simulink model "TGASMODEL"  (R2021b)
settings: Solver=VariableStepAuto  StartTime=0.0  StopTime=simstoptime  RelTol=1e-3
values from neighbouring files (symbols this model uses):
  initial_lane = 0    [setupscript.m]
  Ts = 0.1    [setupscript.m]
  v_set = 33    [setupscript.m]
  VB = 30.5556    [setupscript.m]
  velocity_left_lane_max = 35    [setupscript.m]
  velocity_right_lane_max = 35    [setupscript.m]
undefined symbols (not defined in the file or in its folder): driving
libraries: drivingscenarioandsensors x3, autolibshared x1
settings Model: Creator=Milin  LastModifiedBy=Milin.Patel
settings SolverCC: AlgebraicLoopSolver=TrustRegion
settings DebuggingCC: ParameterPrecisionLossMsg=none  SFMachineParentedDataDiag=warning

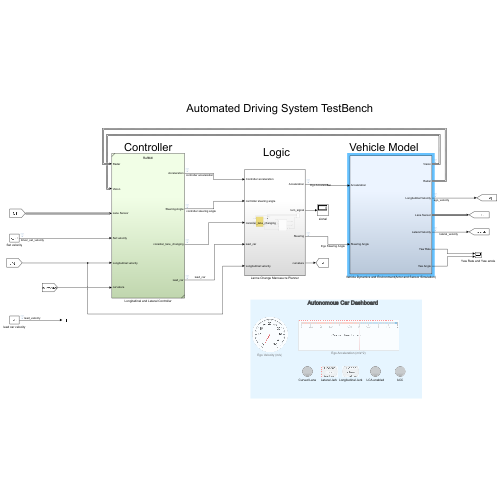
[thumbnail: Simulink's stored preview of the top-level diagram]
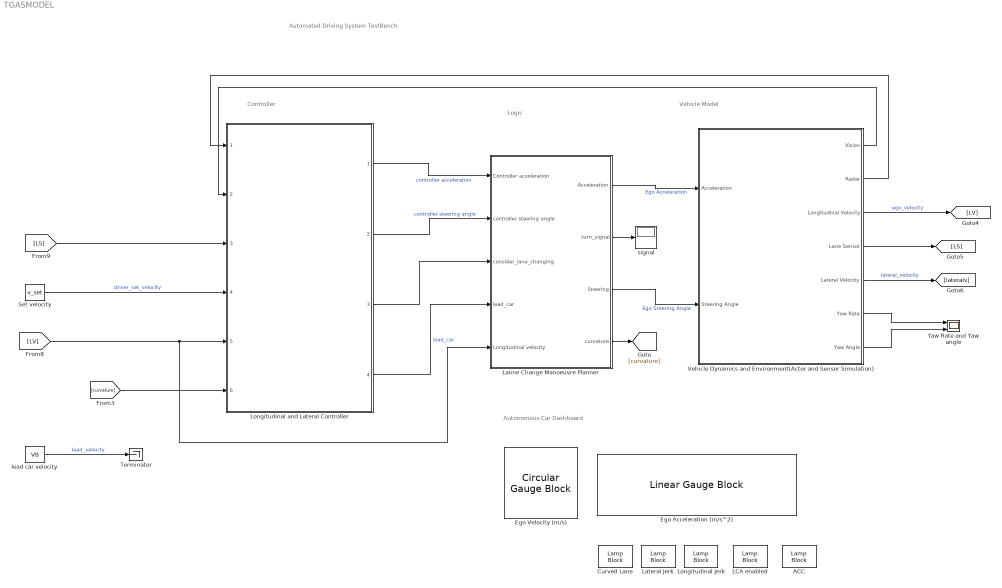
== system TGASMODEL ==
  note: Autonomous Car Dashboard
  note: Automated Driving System TestBench
  note: Controller
  note: Vehicle Model
  note: Logic
  ACC : LampBlock  LabelPosition=Hide
  Curved Lane : LampBlock  LabelPosition=Hide
  Ego Acceleration (m/s^2) : LinearGaugeBlock  LabelPosition=Hide  ScaleMin=-3  ScaleMax=2
  Ego Velocity (m/s) : CircularGaugeBlock  LabelPosition=Hide  ScaleMax=50  TickInterval=5
  LCA enabled : LampBlock  LabelPosition=Hide
  Lanne Change Manoeuvre Planner : Subsystem
  Lateral Jerk : LampBlock  LabelPosition=Hide
  Longitudinal Jerk : LampBlock  LabelPosition=Hide
  Longitudinal and Lateral Controller : Subsystem  ReferencedSubsystem=RefMdl
  Set velocity : Constant  Value=v_set  SampleTime=Ts
  Terminator : Terminator
  Vehicle Dynamics and Environment(Actor and Sensor Simulation) : Subsystem
  Yaw Rate and Yaw angle : Scope  NumInputPorts=2
  lead car velocity : Constant  Value=VB  SampleTime=Ts
  signal : Display
  wires:
  Vehicle Dynamics and Environment(Actor and Sensor Simulation)/3(Longitudinal Velocity) -> [LV]  "ego_velocity"
  Vehicle Dynamics and Environment(Actor and Sensor Simulation)/7(Yaw Angle) -> Yaw Rate and Yaw angle/2
  Vehicle Dynamics and Environment(Actor and Sensor Simulation)/4(Lane Sensor) -> [LS]
  Longitudinal and Lateral Controller/2 -> Lanne Change Manoeuvre Planner/2(controller steering angle)  "controller steering angle"
  Lanne Change Manoeuvre Planner/1(Acceleration) -> Vehicle Dynamics and Environment(Actor and Sensor Simulation)/1(Acceleration)  "Ego Acceleration"
  Vehicle Dynamics and Environment(Actor and Sensor Simulation)/6(Yaw Rate) -> Yaw Rate and Yaw angle/1
  Lanne Change Manoeuvre Planner/2(turn_signal) -> signal/1
  Vehicle Dynamics and Environment(Actor and Sensor Simulation)/1(Vision) -> Longitudinal and Lateral Controller/2
  Vehicle Dynamics and Environment(Actor and Sensor Simulation)/2(Radar) -> Longitudinal and Lateral Controller/1
  [LS] -> Longitudinal and Lateral Controller/3
  Longitudinal and Lateral Controller/3 -> Lanne Change Manoeuvre Planner/3(consider_lane_changing)
  Lanne Change Manoeuvre Planner/4(curvature) -> [curvature]
  Lanne Change Manoeuvre Planner/3(Steering) -> Vehicle Dynamics and Environment(Actor and Sensor Simulation)/2(Steering Angle)  "Ego Steering Angle"
  [curvature] -> Longitudinal and Lateral Controller/6
  Set velocity/1 -> Longitudinal and Lateral Controller/4  "driver_set_velocity"
  Longitudinal and Lateral Controller/1 -> Lanne Change Manoeuvre Planner/1(Controller acceleration)  "controller acceleration"
  Vehicle Dynamics and Environment(Actor and Sensor Simulation)/5(Lateral Velocity) -> [lateralv]  "lateral_velocity"
  [LV] -> Lanne Change Manoeuvre Planner/5(Longitudinal velocity), Longitudinal and Lateral Controller/5
  lead car velocity/1 -> Terminator/1  "lead_velocity"
  Longitudinal and Lateral Controller/4 -> Lanne Change Manoeuvre Planner/4(lead_car)  "lead_car"

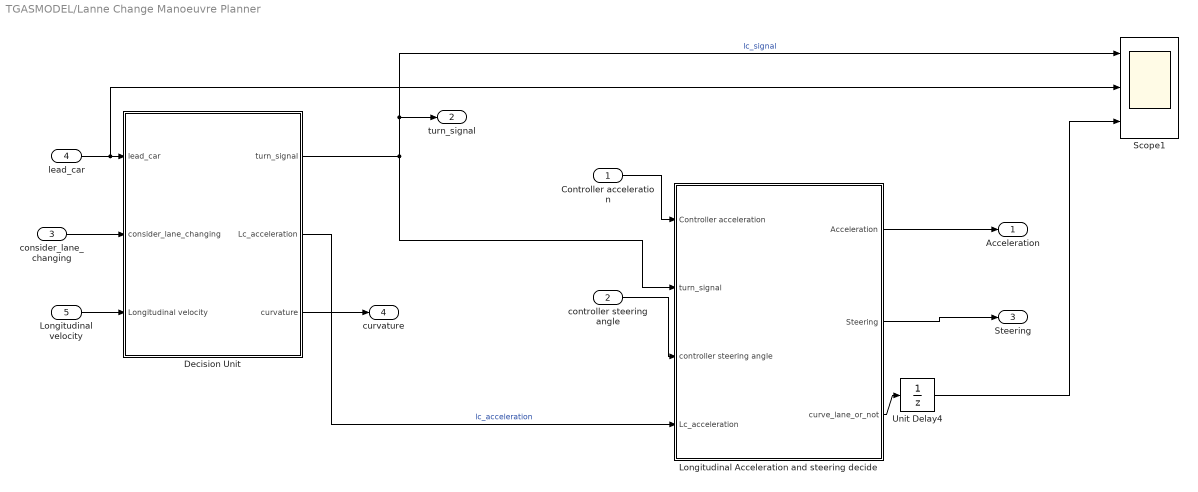
== system TGASMODEL/Lanne Change Manoeuvre Planner ==
  Controller acceleration : Inport
  controller steering angle : Inport  Port=2
  consider_lane_changing : Inport  Port=3
  lead_car : Inport  Port=4
  Longitudinal velocity : Inport  Port=5
  Decision Unit : Subsystem
  Longitudinal Acceleration and steering decide : Subsystem
  Scope1 : Scope  NumInputPorts=3
  Unit Delay4 : UnitDelay  SampleTime=-1  HasFrameUpgradeWarning=on
  Acceleration : Outport
  turn_signal : Outport  Port=2
  Steering : Outport  Port=3
  curvature : Outport  Port=4
  wires:
  consider_lane_changing/1 -> Decision Unit/2(consider_lane_changing)
  controller steering angle/1 -> Longitudinal Acceleration and steering decide/3(controller steering angle)
  Controller acceleration/1 -> Longitudinal Acceleration and steering decide/1(Controller acceleration)
  Longitudinal velocity/1 -> Decision Unit/3(Longitudinal velocity)
  lead_car/1 -> Scope1/2, Decision Unit/1(lead_car)
  Decision Unit/1(turn_signal) -> Scope1/1, turn_signal/1, Longitudinal Acceleration and steering decide/2(turn_signal)  "lc_signal"
  Decision Unit/3(curvature) -> curvature/1
  Decision Unit/2(Lc_acceleration) -> Longitudinal Acceleration and steering decide/4(Lc_acceleration)  "lc_acceleration"
  Longitudinal Acceleration and steering decide/1(Acceleration) -> Acceleration/1
  Longitudinal Acceleration and steering decide/2(Steering) -> Steering/1
  Unit Delay4/1 -> Scope1/3
  Longitudinal Acceleration and steering decide/3(curve_lane_or_not) -> Unit Delay4/1

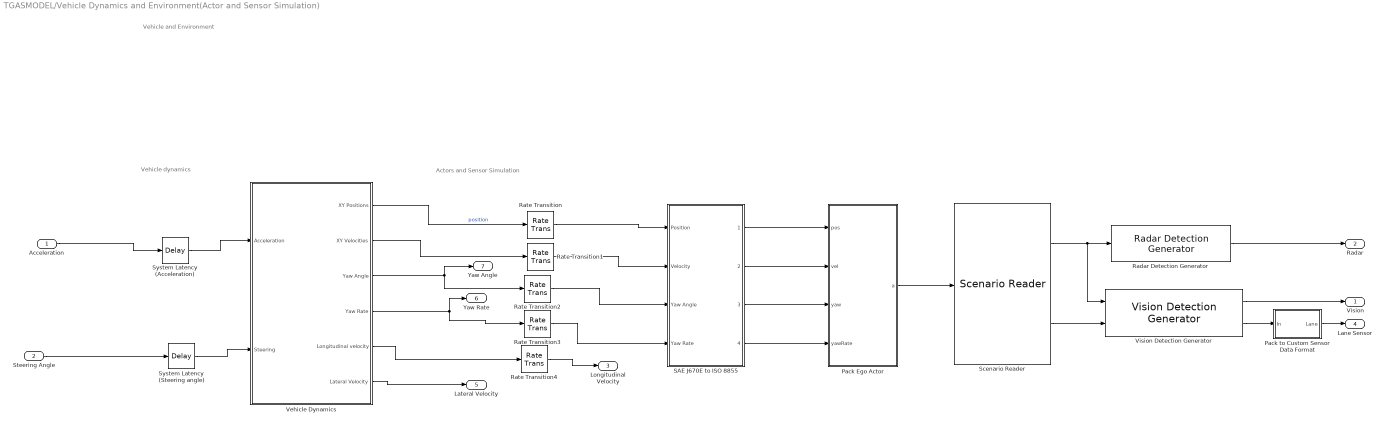
== system TGASMODEL/Vehicle Dynamics and Environment(Actor and Sensor Simulation) ==
  note: Vehicle dynamics
  note: Actors and Sensor Simulation
  note: Vehicle and Environment
  Acceleration : Inport  Unit=m/s^2
  Steering Angle : Inport  Port=2  Unit=rad
  Pack Ego Actor : MATLAB Function  TreatAsAtomicUnit=on
  Pack to Custom Sensor Data Format : Subsystem
  Radar Detection Generator : drivingscenarioandsensors/Radar Detection Generator  SensorIndex=2  UpdateInterval=0.1  SensorLocation=[ 3.7, 0 ]  Height=0.2  Yaw=0  Pitch=0  Roll=0  BusNameSource=Property  BusName=BusRadar  MaxNumDetectionsSource=Property  MaxNumDetections=50  DetectionCoordinates=Ego Cartesian  SimulateUsing=Interpreted execution  AzimuthResolution=4  ElevationResolution=10  RangeResolution=2.5  RangeRateResolution=0.5  AzimuthBiasFraction=0.1  ElevationBiasFraction=0.1  RangeBiasFraction=0.05  RangeRateBiasFraction=0.05  FieldOfView=[ 20, 5 ]  MaxRange=174  RangeRateLimits=[ -100, 100 ]  DetectionProbability=0.9  FalseAlarmRate=1e-6  ReferenceRange=100  ReferenceRCS=0  HasElevation=off  HasRangeRate=on  HasNoise=on  HasFalseAlarms=on  HasOcclusion=on  InitialSeedSource=Repeatable  InitialSeed=0  UsedSeed=driving.internal.SimulinkUtilities.seedManager(gcb)  ActorProfilesSource=MATLAB expression  ActorProfilesParameters=driving.internal.ActorProfilesRadarParameters  ActorProfilesExpression=actor_Profiles
      settings: SourceProductBaseCode=DR
  Rate Transition{,1..4} (5 alike) : RateTransition  OutPortSampleTime=Ts
  SAE J670E to ISO 8855 : Subsystem
  Scenario Reader : drivingscenarioandsensors/Scenario Reader  ScenarioSource=From file  ScenarioFileName=D:\Simulations\Thesis submission digital files\Thesis submission digital files\TGAS Model Testbench\customlc.mat  ScenarioVariableName=scenario  OutputCoordinateSystem=Vehicle coordinates  EgoVehicleSource=Input port  EgoVehicleActorID=1  OrientVehiclesOnRoad=off  OutputEgoVehiclePose=off  OutputEgoVehicleState=off  SampleTime=0.1  LaneBoundaryOutput=Ego vehicle lane boundaries  LaneBoundaryDistance=0:0.5:60  LaneBoundaryLocation=Inner edge of lane markings  BusNameSource=Auto  BusName=BusActors1  BusNumActorsSource=Scenario  BusNumActors=100  BusName2Source=Auto  BusName2=BusLaneBoundaries  BusNumLaneBoundariesSource=Scenario  BusNumLaneBoundaries=10  BusName3Source=Auto  BusName3=BusEgoActor  BusName4Source=Auto  BusName4=BusEgoState  ShowCoordinateLabels=on  SimulateUsing=Interpreted execution
  System Latency (Acceleration) : TransportDelay  DelayTime=Ts  BufferSize=2048
  System Latency (Steering angle) : TransportDelay  DelayTime=Ts  BufferSize=2048
  Vehicle Dynamics : Subsystem  VariantControl=Variant2
  Vision Detection Generator : drivingscenarioandsensors/Vision Detection Generator  SensorIndex=1  DetectorOutput=Lanes and objects  UpdateInterval=0.1  LaneUpdateInterval=0.1  SensorLocation=[ 1.9, 0 ]  Height=1.1  Yaw=0  Pitch=1  Roll=0  BusNameSource=Property  BusName=BusVision  BusName2Source=Property  BusName2=BusLanes  MaxNumDetectionsSource=Property  MaxNumDetections=20  MaxNumLanesSource=Property  MaxNumLanes=2  DetectionCoordinates=Ego Cartesian  SimulateUsing=Interpreted execution  MaxRange=150  BoundingBoxAccuracy=5  ProcessNoiseIntensity=5  MaxSpeed=50  MaxAllowedOcclusion=0.5  MinObjectImageSize=[ 10, 10 ]  DetectionProbability=0.9  FalsePositivesPerImage=0.1  MinLaneImageSize=[ 20, 3 ]  LaneBoundaryAccuracy=3  HasNoise=on  InitialSeedSource=Repeatable  InitialSeed=0  UsedSeed=driving.internal.SimulinkUtilities.seedManager(gcb)  ActorProfilesSource=MATLAB expression  ActorProfilesParameters=driving.internal.ActorProfilesParameters  ActorProfilesExpression=actor_Profiles  Intrinsics=driving.internal.cameraIntrinsics('FocalLength',[ 800,800 ])
  Vision : Outport  VectorParamsAs1DForOutWhenUnconnected=off
  Radar : Outport  Port=2  VectorParamsAs1DForOutWhenUnconnected=off
  Longitudinal Velocity : Outport  Port=3  VectorParamsAs1DForOutWhenUnconnected=off
  Lane Sensor : Outport  Port=4  VectorParamsAs1DForOutWhenUnconnected=off
  Lateral Velocity : Outport  Port=5  VectorParamsAs1DForOutWhenUnconnected=off
  Yaw Rate : Outport  Port=6
  Yaw Angle : Outport  Port=7
  wires:
  Scenario Reader/1 -> Vision Detection Generator/1, Radar Detection Generator/1
  Vehicle Dynamics/2(XY Velocities) -> Rate Transition1/1
  Vehicle Dynamics/1(XY Positions) -> Rate Transition/1  "position"
  Scenario Reader/2 -> Vision Detection Generator/2
  Vision Detection Generator/1 -> Vision/1
  Radar Detection Generator/1 -> Radar/1
  Pack Ego Actor/1(a) -> Scenario Reader/1
  Acceleration/1 -> System Latency (Acceleration)/1
  Steering Angle/1 -> System Latency (Steering angle)/1
  System Latency (Acceleration)/1 -> Vehicle Dynamics/1(Acceleration)
  System Latency (Steering angle)/1 -> Vehicle Dynamics/2(Steering)
  SAE J670E to ISO 8855/1(1) -> Pack Ego Actor/1(pos)
  SAE J670E to ISO 8855/2(2) -> Pack Ego Actor/2(vel)
  SAE J670E to ISO 8855/3(3) -> Pack Ego Actor/3(yaw)
  SAE J670E to ISO 8855/4(4) -> Pack Ego Actor/4(yawRate)
  Rate Transition3/1 -> SAE J670E to ISO 8855/4(Yaw Rate)
  Rate Transition2/1 -> SAE J670E to ISO 8855/3(Yaw Angle)
  Rate Transition1/1 -> SAE J670E to ISO 8855/2(Velocity)
  Rate Transition/1 -> SAE J670E to ISO 8855/1(Position)
  Vehicle Dynamics/6(Lateral Velocity) -> Lateral Velocity/1
  Vehicle Dynamics/3(Yaw Angle) -> Yaw Angle/1, Rate Transition2/1
  Vehicle Dynamics/4(Yaw Rate) -> Yaw Rate/1, Rate Transition3/1
  Vehicle Dynamics/5(Longitudinal velocity) -> Rate Transition4/1
  Rate Transition4/1 -> Longitudinal Velocity/1
  Vision Detection Generator/2 -> Pack to Custom Sensor Data Format/1(In)
  Pack to Custom Sensor Data Format/1("Lane ") -> Lane Sensor/1

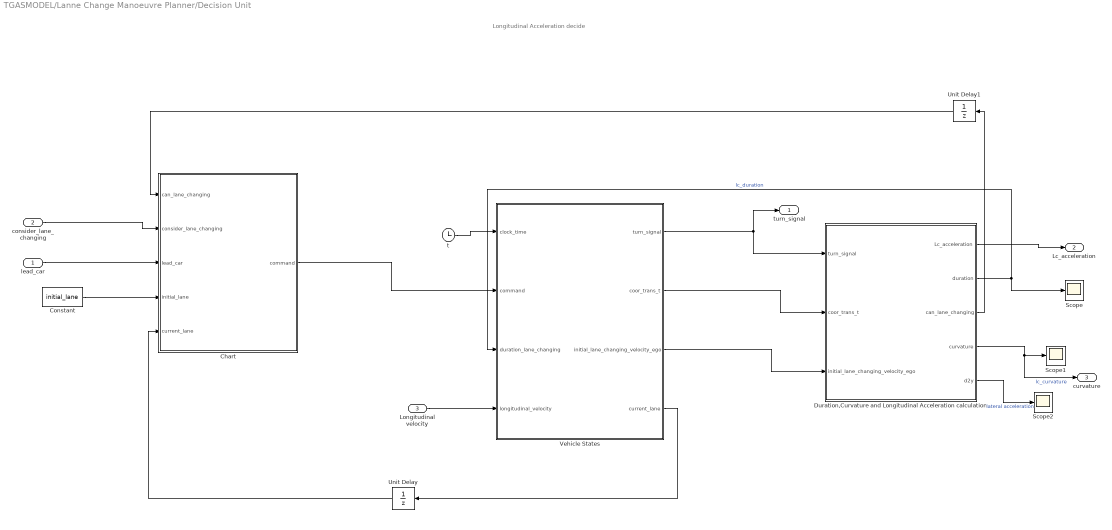
== system TGASMODEL/Lanne Change Manoeuvre Planner/Decision Unit ==
  note: Longitudinal Acceleration decide
  lead_car : Inport
  consider_lane_changing : Inport  Port=2
  Longitudinal velocity : Inport  Port=3
  Chart : Stateflow chart  TreatAsAtomicUnit=on
  Constant : Constant  Value=initial_lane
  Duration,Curvature and Longitudinal Acceleration calculation : Subsystem
  Scope : Scope
  Scope1 : Scope
  Scope2 : Scope
  Unit Delay : UnitDelay  SampleTime=-1  HasFrameUpgradeWarning=on
  Unit Delay1 : UnitDelay  SampleTime=-1  HasFrameUpgradeWarning=on
  Vehicle States : Stateflow chart  TreatAsAtomicUnit=on
      settings: PortSchema="{\"entries\":[{\"content\":{\"sides\":[{\"content\":{\"connectorIds\":[\"In2\",\"In1\",\"In3\",\"In4\"]},\"type\":\"ConnectorPlacement.EquallySpacedRectSide\",\"uuid\":\"633906ca-579d-4042-9cc9-7aca433b340e\"},{\"content\":{\"connectorIds\":[\"Out1\",\"Out2\",\"Out3\",\"Out4\"],\"side\":\"RIGHT\"},\"type\":\"ConnectorPlacement.EquallySpacedRectSide\",\"uuid\":\"b2f4b13f-832c-4f85-a2c3-5544fdd2b38b\"},{\"content\":{\"connectorIds\":[],\"side\":\"TOP\"},\"type\":\"ConnectorPlacement.EquallySpacedRectSide\",\"uuid\":\"a13a6fde-8974-48e1-9856-53eff330f07d\"}]},\"type\":\"ConnectorPlacement.EquallySpacedConnector\",\"uuid\":\"3aa8cc94-316d-4e92-871e-4708a17b4e4c\"}],\"packageUris\":[\"http://schema.mathworks.com/mf0/Connector/R2020b\"],\"version\":\"1.0\"}"
  t : Clock
  turn_signal : Outport
  Lc_acceleration : Outport  Port=2
  curvature : Outport  Port=3
  wires:
  Vehicle States/1(turn_signal) -> Duration,Curvature and Longitudinal Acceleration calculation/1(turn_signal), turn_signal/1
  t/1 -> Vehicle States/2(clock_time)
  Vehicle States/3(initial_lane_changing_velocity_ego) -> Duration,Curvature and Longitudinal Acceleration calculation/3(initial_lane_changing_velocity_ego)
  Duration,Curvature and Longitudinal Acceleration calculation/1(Lc_acceleration) -> Lc_acceleration/1
  Duration,Curvature and Longitudinal Acceleration calculation/2(duration) -> Scope/1, Vehicle States/3(duration_lane_changing)  "lc_duration"
  Duration,Curvature and Longitudinal Acceleration calculation/4(curvature) -> curvature/1, Scope1/1  "lc_curvature"
  Longitudinal velocity/1 -> Vehicle States/4(longitudinal_velocity)
  Vehicle States/2(coor_trans_t) -> Duration,Curvature and Longitudinal Acceleration calculation/2(coor_trans_t)
  lead_car/1 -> Chart/3(lead_car)
  consider_lane_changing/1 -> Chart/2(consider_lane_changing)
  Constant/1 -> Chart/4(initial_lane)
  Chart/1(command) -> Vehicle States/1(command)
  Vehicle States/4(current_lane) -> Unit Delay/1
  Unit Delay/1 -> Chart/5(current_lane)
  Duration,Curvature and Longitudinal Acceleration calculation/3(can_lane_changing) -> Unit Delay1/1
  Unit Delay1/1 -> Chart/1(can_lane_changing)
  Duration,Curvature and Longitudinal Acceleration calculation/5(d2y) -> Scope2/1  "lateral acceleration"

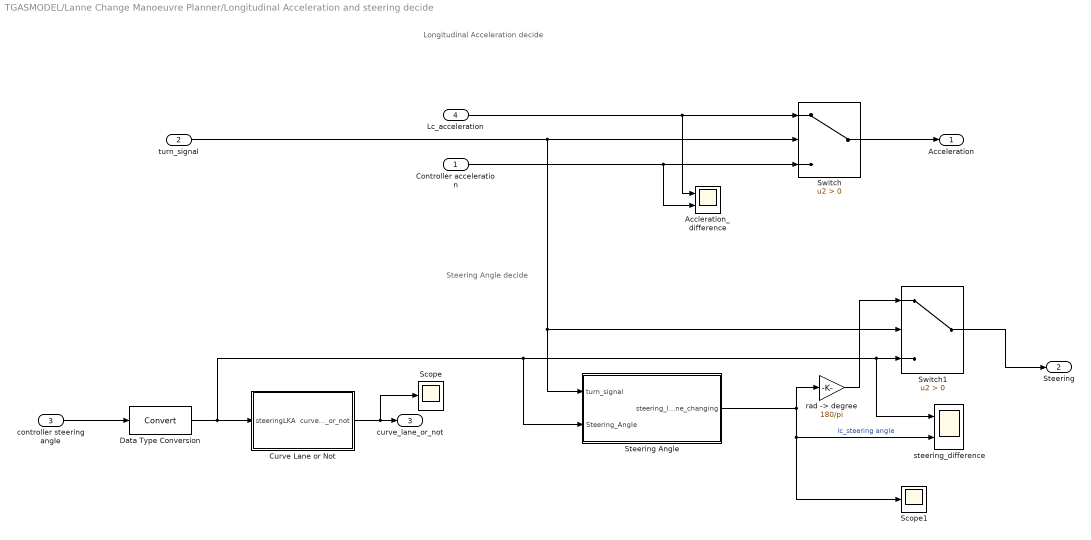
== system TGASMODEL/Lanne Change Manoeuvre Planner/Longitudinal Acceleration and steering decide ==
  note: Steering Angle decide
  note: Longitudinal Acceleration decide
  Controller acceleration : Inport
  turn_signal : Inport  Port=2
  controller steering angle : Inport  Port=3
  Lc_acceleration : Inport  Port=4
  Accleration_difference : Scope  NumInputPorts=2
  Curve Lane or Not : MATLAB Function  TreatAsAtomicUnit=on
  Data Type Conversion : DataTypeConversion
  Scope : Scope
  Scope1 : Scope
  "Steering Angle " : MATLAB Function  TreatAsAtomicUnit=on
  Switch : Switch  Criteria=u2 > Threshold
  Switch1 : Switch  Criteria=u2 > Threshold
  "rad -> degree" : Gain  Gain=180/pi
  steering_difference : Scope  NumInputPorts=2
  Acceleration : Outport
  Steering : Outport  Port=2
  curve_lane_or_not : Outport  Port=3
  wires:
  Lc_acceleration/1 -> Accleration_difference/1, Switch/1
  turn_signal/1 -> Switch/2, "Steering Angle "/1(turn_signal), Switch1/2
  Controller acceleration/1 -> Switch/3, Accleration_difference/2
  Switch/1 -> Acceleration/1
  Switch1/1 -> Steering/1
  Data Type Conversion/1 -> "Steering Angle "/2(Steering_Angle), steering_difference/1, Switch1/3, Curve Lane or Not/1(steeringLKA)
  Curve Lane or Not/1(curve_lane_or_not) -> curve_lane_or_not/1, Scope/1
  controller steering angle/1 -> Data Type Conversion/1
  "rad -> degree"/1 -> Switch1/1
  "Steering Angle "/1(steering_lane_changing) -> "rad -> degree"/1, steering_difference/2, Scope1/1  "lc_steering angle"

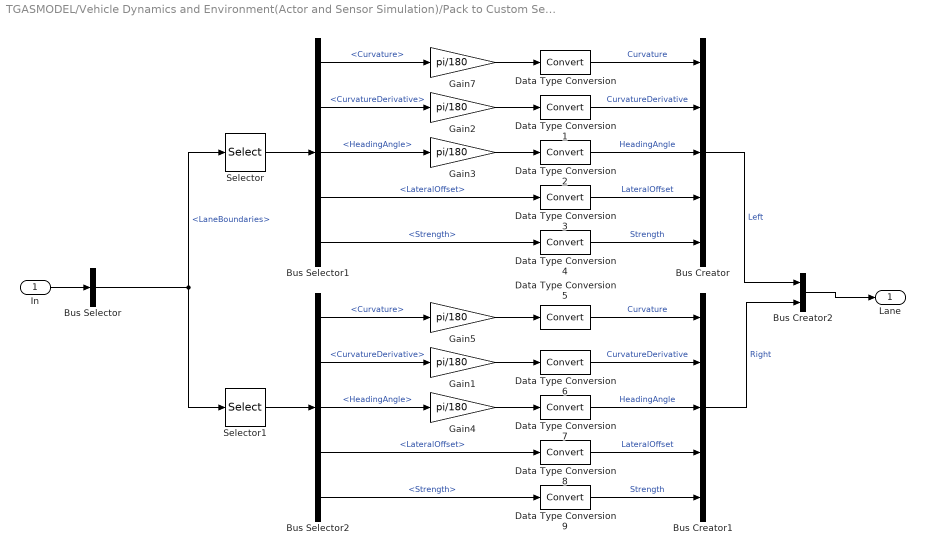
== system TGASMODEL/Vehicle Dynamics and Environment(Actor and Sensor Simulation)/Pack to Custom Sensor Data Format ==
  In : Inport
  Bus Creator : BusCreator  Inputs=5  OutDataTypeStr=Bus: LaneSensorBoundaries
  Bus Creator1 : BusCreator  Inputs=5  OutDataTypeStr=Bus: LaneSensorBoundaries
  Bus Creator2 : BusCreator  Inputs=2  OutDataTypeStr=Bus: LaneSensor
  Bus Selector : BusSelector  OutputSignals=LaneBoundaries
  Bus Selector1 : BusSelector  OutputSignals=Curvature,CurvatureDerivative,HeadingAngle,LateralOffset,Strength
  Bus Selector2 : BusSelector  OutputSignals=Curvature,CurvatureDerivative,HeadingAngle,LateralOffset,Strength
  Data Type Conversion{,1..9} (10 alike) : DataTypeConversion
  Gain{1..5,7} (6 alike) : Gain  Gain=pi/180
  Selector : Selector  InputPortWidth=2  IndexOptions=Index vector (dialog)  Indices=1  OutputSizes=1
  Selector1 : Selector  InputPortWidth=2  IndexOptions=Index vector (dialog)  Indices=2  OutputSizes=1
  "Lane " : Outport  VectorParamsAs1DForOutWhenUnconnected=off
  wires:
  In/1 -> Bus Selector/1
  Bus Selector/1 -> Selector/1, Selector1/1  "<LaneBoundaries>"
  Selector/1 -> Bus Selector1/1
  Bus Selector1/2 -> Gain2/1  "<CurvatureDerivative>"
  Bus Selector1/1 -> Gain7/1  "<Curvature>"
  Bus Selector1/3 -> Gain3/1  "<HeadingAngle>"
  Gain7/1 -> Data Type Conversion/1
  Gain2/1 -> Data Type Conversion1/1
  Gain3/1 -> Data Type Conversion2/1
  Bus Selector1/4 -> Data Type Conversion3/1  "<LateralOffset>"
  Bus Selector1/5 -> Data Type Conversion4/1  "<Strength>"
  Data Type Conversion/1 -> Bus Creator/1  "Curvature"
  Data Type Conversion1/1 -> Bus Creator/2  "CurvatureDerivative"
  Data Type Conversion2/1 -> Bus Creator/3  "HeadingAngle"
  Data Type Conversion3/1 -> Bus Creator/4  "LateralOffset"
  Data Type Conversion4/1 -> Bus Creator/5  "Strength"
  Data Type Conversion9/1 -> Bus Creator1/5  "Strength"
  Data Type Conversion6/1 -> Bus Creator1/2  "CurvatureDerivative"
  Data Type Conversion7/1 -> Bus Creator1/3  "HeadingAngle"
  Data Type Conversion8/1 -> Bus Creator1/4  "LateralOffset"
  Data Type Conversion5/1 -> Bus Creator1/1  "Curvature"
  Bus Selector2/1 -> Gain5/1  "<Curvature>"
  Selector1/1 -> Bus Selector2/1
  Bus Selector2/4 -> Data Type Conversion8/1  "<LateralOffset>"
  Bus Selector2/5 -> Data Type Conversion9/1  "<Strength>"
  Bus Selector2/2 -> Gain1/1  "<CurvatureDerivative>"
  Gain4/1 -> Data Type Conversion7/1
  Gain5/1 -> Data Type Conversion5/1
  Gain1/1 -> Data Type Conversion6/1
  Bus Selector2/3 -> Gain4/1  "<HeadingAngle>"
  Bus Creator2/1 -> "Lane "/1
  Bus Creator/1 -> Bus Creator2/1  "Left"
  Bus Creator1/1 -> Bus Creator2/2  "Right"

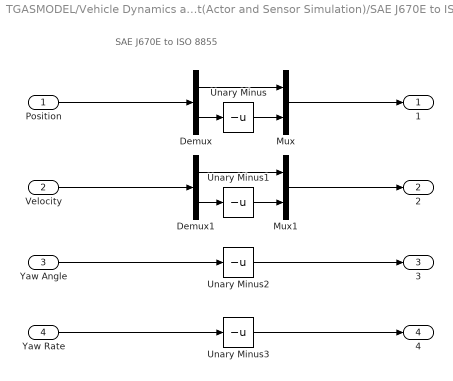
== system TGASMODEL/Vehicle Dynamics and Environment(Actor and Sensor Simulation)/SAE J670E to ISO 8855 ==
  note: SAE J670E to ISO 8855
  Position : Inport  Unit=m
  Velocity : Inport  Port=2  Unit=m/s
  Yaw Angle : Inport  Port=3  Unit=deg
  Yaw Rate : Inport  Port=4  Unit=deg/s
  Demux : Demux  Outputs=2
  Demux1 : Demux  Outputs=2
  Mux : Mux  Inputs=2
  Mux1 : Mux  Inputs=2
  Unary Minus{,1..3} (4 alike) : UnaryMinus
  1 : Outport  VectorParamsAs1DForOutWhenUnconnected=off
  2 : Outport  Port=2  VectorParamsAs1DForOutWhenUnconnected=off
  3 : Outport  Port=3  VectorParamsAs1DForOutWhenUnconnected=off
  4 : Outport  Port=4  VectorParamsAs1DForOutWhenUnconnected=off
  wires:
  Yaw Rate/1 -> Unary Minus3/1
  Yaw Angle/1 -> Unary Minus2/1
  Demux/1 -> Mux/1
  Demux/2 -> Unary Minus/1
  Unary Minus/1 -> Mux/2
  Unary Minus1/1 -> Mux1/2
  Demux1/2 -> Unary Minus1/1
  Demux1/1 -> Mux1/1
  Mux1/1 -> 2/1
  Mux/1 -> 1/1
  Position/1 -> Demux/1
  Velocity/1 -> Demux1/1
  Unary Minus2/1 -> 3/1
  Unary Minus3/1 -> 4/1

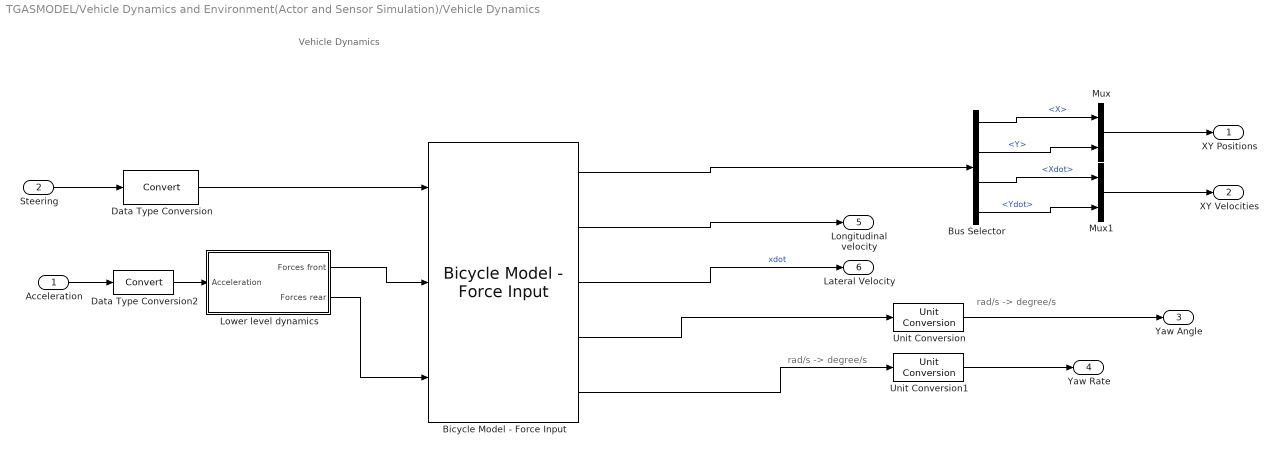
== system TGASMODEL/Vehicle Dynamics and Environment(Actor and Sensor Simulation)/Vehicle Dynamics ==
  note: rad/s -> degree/s
  note: Vehicle Dynamics
  note: rad/s -> degree/s
  Acceleration : Inport  Unit=m/s^2
  Steering : Inport  Port=2  Unit=rad
  Bicycle Model - Force Input : autolibshared/Bicycle Model - Force Input  trackMode=Single (bicycle)  inputMode=External longitudinal forces  frontSteerMode=on  rearSteerMode=off  windMode=off  muMode=off  extFMode=off  extMMode=off  aMode=3  NF=2  NR=2  m=1575  a=1.2  b=1.6  h=0.35  X_o=x0_ego  xdot_o=v0_ego  CalphaMode=off  sigmaMode=on  w=[1.4,1.4]  Cy_f=19000  Cy_r=33000  sigma_f=.1  sigma_r=.1  alpha_f_brk=[-.1 .1]  Cy_f_data=[-9e3 9e3]  alpha_r_brk=[-.1 .1]  Cy_r_data=[-9e3 9e3]  Y_o=y0_ego  ydot_o=0  Izz=2875  psi_o=0  r_o=0  Af=0  Cd=.3  Cl=.1  Cpm=.1  beta_w=[0:0.01:0.3]  Cs=[0:0.03:0.9]  Cym=[0:0.01:0.3]  Pabs=101325  Tair=273  g=9.81  mu=1  xdot_tol=.01  Fznom=5000  Fxtire_sat=1e6  Fytire_sat=1e6  longOff=0  latOff=0  vertOff=0
      settings: SourceProductBaseCode=PW,DR,MT,UV,VE
  Bus Selector : BusSelector  OutputSignals=InertFrm.FrntAxl.Disp.X,InertFrm.FrntAxl.Disp.Y,InertFrm.FrntAxl.Vel.Xdot,InertFrm.FrntAxl.Vel.Ydot
  Data Type Conversion : DataTypeConversion
  Data Type Conversion2 : DataTypeConversion
  Lower level dynamics : Subsystem
  Mux : Mux  Inputs=2
  Mux1 : Mux  Inputs=2
  Unit Conversion : UnitConversion  OutputType=Inherit: Inherit via back propagation
  Unit Conversion1 : UnitConversion  OutputType=Inherit: Inherit via back propagation
  XY Positions : Outport  Unit=m  VectorParamsAs1DForOutWhenUnconnected=off
  XY Velocities : Outport  Port=2  Unit=m/s  VectorParamsAs1DForOutWhenUnconnected=off
  Yaw Angle : Outport  Port=3  Unit=deg  VectorParamsAs1DForOutWhenUnconnected=off
  Yaw Rate : Outport  Port=4  Unit=degree/s  VectorParamsAs1DForOutWhenUnconnected=off
  Longitudinal velocity : Outport  Port=5  VectorParamsAs1DForOutWhenUnconnected=off
  Lateral Velocity : Outport  Port=6
  wires:
  Data Type Conversion2/1 -> Lower level dynamics/1(Acceleration)
  Acceleration/1 -> Data Type Conversion2/1
  Lower level dynamics/2(Forces rear) -> Bicycle Model - Force Input/3
  Lower level dynamics/1(Forces front) -> Bicycle Model - Force Input/2
  Bicycle Model - Force Input/3 -> Lateral Velocity/1  "xdot"
  Bus Selector/1 -> Mux/1  "<X>"
  Unit Conversion1/1 -> Yaw Rate/1
  Bicycle Model - Force Input/2 -> Longitudinal velocity/1
  Bus Selector/2 -> Mux/2  "<Y>"
  Bus Selector/4 -> Mux1/2  "<Ydot>"
  Mux1/1 -> XY Velocities/1
  Bus Selector/3 -> Mux1/1  "<Xdot>"
  Mux/1 -> XY Positions/1
  Bicycle Model - Force Input/1 -> Bus Selector/1
  Unit Conversion/1 -> Yaw Angle/1
  Bicycle Model - Force Input/4 -> Unit Conversion/1
  Bicycle Model - Force Input/5 -> Unit Conversion1/1
  Steering/1 -> Data Type Conversion/1
  Data Type Conversion/1 -> Bicycle Model - Force Input/1

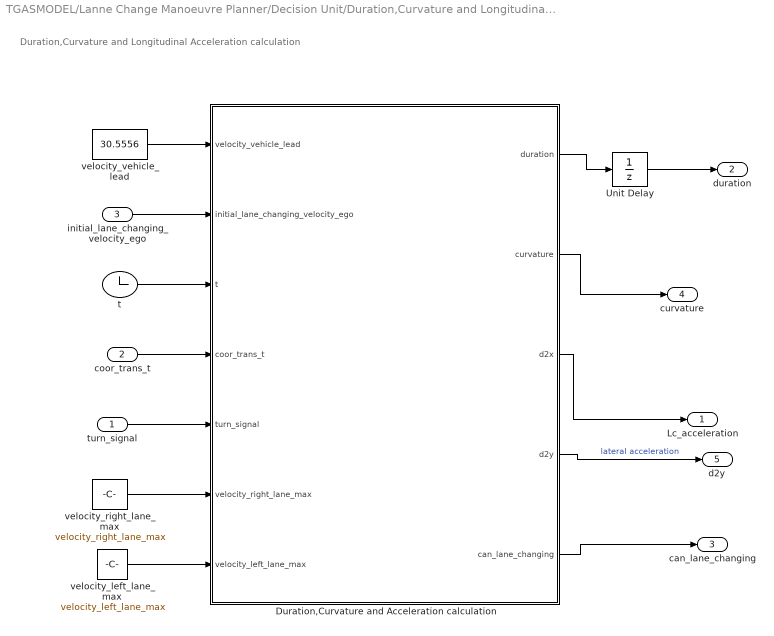
== system TGASMODEL/Lanne Change Manoeuvre Planner/Decision Unit/Duration,Curvature and Longitudinal Acceleration calculation ==
  note: Duration,Curvature and Longitudinal Acceleration calculation
  turn_signal : Inport
  coor_trans_t : Inport  Port=2
  initial_lane_changing_velocity_ego : Inport  Port=3
  Duration,Curvature and Acceleration calculation : MATLAB Function  TreatAsAtomicUnit=on
  Unit Delay : UnitDelay  SampleTime=-1  HasFrameUpgradeWarning=on
  t : Clock
  velocity_left_lane_max : Constant  Value=velocity_left_lane_max
  velocity_right_lane_max : Constant  Value=velocity_right_lane_max
  velocity_vehicle_lead : Constant  Value=30.5556
  Lc_acceleration : Outport
  duration : Outport  Port=2
  can_lane_changing : Outport  Port=3
  curvature : Outport  Port=4
  d2y : Outport  Port=5
  wires:
  velocity_left_lane_max/1 -> Duration,Curvature and Acceleration calculation/7(velocity_left_lane_max)
  t/1 -> Duration,Curvature and Acceleration calculation/3(t)
  Duration,Curvature and Acceleration calculation/3(d2x) -> Lc_acceleration/1
  Duration,Curvature and Acceleration calculation/1(duration) -> Unit Delay/1
  Duration,Curvature and Acceleration calculation/2(curvature) -> curvature/1
  initial_lane_changing_velocity_ego/1 -> Duration,Curvature and Acceleration calculation/2(initial_lane_changing_velocity_ego)
  turn_signal/1 -> Duration,Curvature and Acceleration calculation/5(turn_signal)
  Duration,Curvature and Acceleration calculation/5(can_lane_changing) -> can_lane_changing/1
  velocity_right_lane_max/1 -> Duration,Curvature and Acceleration calculation/6(velocity_right_lane_max)
  Unit Delay/1 -> duration/1
  coor_trans_t/1 -> Duration,Curvature and Acceleration calculation/4(coor_trans_t)
  velocity_vehicle_lead/1 -> Duration,Curvature and Acceleration calculation/1(velocity_vehicle_lead)
  Duration,Curvature and Acceleration calculation/4(d2y) -> d2y/1  "lateral acceleration"

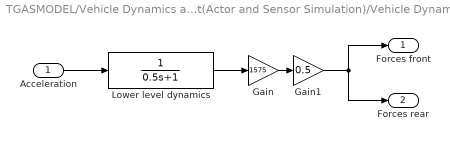
== system TGASMODEL/Vehicle Dynamics and Environment(Actor and Sensor Simulation)/Vehicle Dynamics/Lower level dynamics ==
  Acceleration : Inport
  Gain : Gain  Gain=1575
  Gain1 : Gain  Gain=0.5
  Lower level dynamics : TransferFcn  Denominator=[0.5 1]
  Forces front : Outport  VectorParamsAs1DForOutWhenUnconnected=off
  Forces rear : Outport  Port=2  VectorParamsAs1DForOutWhenUnconnected=off
  wires:
  Gain/1 -> Gain1/1
  Gain1/1 -> Forces front/1, Forces rear/1
  Acceleration/1 -> Lower level dynamics/1
  Lower level dynamics/1 -> Gain/1

== matlab function TGASMODEL/Lanne Change Manoeuvre Planner/Decision Unit/Duration,Curvature and Longitudinal Acceleration calculation/Duration,Curvature and Acceleration calculation ==
  data: velocity_vehicle_lead input; duration output; initial_lane_changing_velocity_ego input; t input; coor_trans_t input; turn_signal input; velocity_right_lane_max input; velocity_left_lane_max input; curvature output; d2x output; d2y output; can_lane_changing output
function [duration,curvature,d2x,d2y,can_lane_changing]= getDurationandCurvatureandAcceleration(velocity_vehicle_lead,initial_lane_changing_velocity_ego,t,coor_trans_t,turn_signal,velocity_right_lane_max,velocity_left_lane_max)

% Calculate the desired curvature,longitudinal velocity and duration of lane changing maneuver.

% Inputs:
% velocity_lead_vehicle: speed of the lead vehicle B. Unit: m/s
% safety_distance: safety distance 

% initial_lane_changing_velocity_ego: the initial speed of lane changing maneuver.

% coor_trans_t: the start time of lane changing maneuver,which is used for coordinate transformation.

% turn_signal: 0->lane keeping,1,2->straight lane changing,3,4->curve lane,changing,

% velocity_right_lane_max: maximal speed allowed on the right lane.
% velocity_left_lane_max: maximal speed allowed on the left lane.


% Outputs:
% curvature: the desired curvature of lane changing.
% d2x: the desired longitudinal acceleration of lane changing.
% duration: the duration of lane changing or u-turn maneuver.
% can_lane_changing: 1->lane changing allowed;0->lane chan ging not allowed.

can_lane_changing=1;
% 
% % the value will be set to one until a good condition for lane change is found.
%  lateral_acceleration_max = 4; % maximal lateral acceleration
%  lateral_acceleration_min = -4;% minimal lateral acceleration
%  longitudinal_acceleration_max = 2; % maximal longitudinal acceleration
% %longitudinal_acceleration_min = -2; % minimal longitudinal acceleration
% % % maximum speed allowed on the left/right lane. Unit:m/s.



% Lane change
if turn_signal == 1 || turn_signal == 2   

    % turn_signal = 1:switch left
    % turn_signal = 2:switch right
    
    velocity_lane_max =  velocity_left_lane_max;
    
if turn_signal == 2
     velocity_lane_max =  velocity_right_lane_max;
end

 % straight lane change
    
 % the target speed velocity_ego_target should be greater than the overtaken
    % vehicle speed by at least 20km/h, while respecting the maximum speed 
    % allowed on the left lane, which yields: 
    
  % velocity_ego_target = min(velocity_vehicle_lead+20km/h,velocity_left_lane_max)
  
  % velocity_leftlane_max is the maximum speed allowed on the left lane.
  
  % the vehicle A can not overtake the vehicle B unless its speed is greater than or equal to the overtaken vehicle speed,this yields: 
 
 % velocity_ego_target = max(min(velocity_vehicle_lead+20km/h,velocity_left_lane_max),velocity_ego_initial)
 % https://tel.archives-ouvertes.fr/tel-01727720/file/These_UTC_Alia_Chebly.pdf,page 40,formula (2.32);
    
velocity_ego_target=max(min(velocity_vehicle_lead + 25*1000/3600, velocity_lane_max),initial_lane_changing_velocity_ego);
    
 distance_between_ego_B_initial = 20;
  
  %the distance between the ego vehicle and the overtaken vehicle at the beginning of the lane changing maneuver
  
 safety_distance = 3; % safety_distance: safety distance between the projection 
%     % of the vehicle A on its lane and the position of the vehicle B on that 
    % lane, when A reaches iTS lane;or the distance between vehicle ego and B when ego vehicle finished the returning 
   
    lane_width=3.6;%lane_width   

    % The derive of duration is at page 40,41,part:
    % Respecting safety requirements,formula (2.36)
    % https://tel.archives-ouvertes.fr/tel-01727720/file/These_UTC_Alia_Chebly.pdf
    
%duration= 2; 
 duration = 2*(distance_between_ego_B_initial - safety_distance )/(velocity_ego_target + initial_lane_changing_velocity_ego - 2*velocity_vehicle_lead);

 % https://tel.archives-ouvertes.fr/tel-01727720/file/These_UTC_Alia_Chebly.pdf
    % The derive of duration_lane_changing_min is at page 39,40,part:
    % Respecting the vehicle dynamic constraints,formula (2.25), (2.30)
    
%   duration_lane_changing_min_1 = max(sqrt(5.77*lane_width/lateral_acceleration_max), sqrt(-5.77*lane_width/lateral_acceleration_min));
%   duration_lane_changing_min_2 = (velocity_ego_target - initial_lane_changing_velocity_ego)/(2/3*longitudinal_acceleration_max);
% % 
%     % page 41, formula(2.39)
%     % In order to find a proper duration(the solution space is not empty),the 
%     % minimal duration must less than the maximal duration.If the solution
%     % space is empty,we decide not to change lane.
%     
%     duration_lane_changing_max = duration;
%     
%     if max(duration_lane_changing_min_1,duration_lane_changing_min_2) < duration_lane_changing_max
%          
%         can_lane_changing = 1;
%      
%     else
%          can_lane_changing = 0;
%      end

    t = t - coor_trans_t; 
    
  % coordinate transformation
  % the equation for longitudinal position:
    % x = a0 + a1*t + a2*t^2 + a3*t^3 + a4*t^4
    
% https://tel.archives-ouvertes.fr/tel-01727720/file/These_UTC_Alia_Chebly.pdf
% page 37,formula (2.15);page 38,formula (2.18)
  
    %a0 = 0;
    a1 = initial_lane_changing_velocity_ego;
    % a2 = 0;
    a3 = (velocity_ego_target - initial_lane_changing_velocity_ego)/duration^2;
    a4 = (-a3/(2*duration));

% the equation for lateral position: 
    
% y = b0 + b1*t + b2*t^2 + b3*t^3 + b4*t^4 + b5*t^5
    
% https://tel.archives-ouvertes.fr/tel-01727720/file/These_UTC_Alia_Chebly.pdf
% page 37,formula (2.16);page 38,formula (2.20)

    % b0 = 0;
    % b1 = 0;
    % b2 = 0;
    b3 = 10*lane_width/duration^3;%((-1)^(turn_signal + 1))
    b4 = (-15)*lane_width/duration^4;
    b5 = 6*lane_width/duration^5;

    % Desired x position
    % x = a1*(time)+a3*(time)^3+a4*(time)^4;
    % Desired y position
    % y = b3*(time)^3+b4*(time)^4+b5*(time)^5;

  % Desired curvature;
    % https://en.wikipedia.org/wiki/Curvature
    % part:In terms of a general parametrization
   
 
    dx = a1 + 3*a3*t^2 + 4*a4*t^3;  % longitudinal velocity 
    
    d2x= 6*a3*t + 12*a4*t^2; % longitudinal acceleration 
    
    dy = 3*b3*t^2 + 4*b4*t^3 + 5*b5*t^4; % lateral velocity 
    
    d2y = 6*b3*t + 12*b4*t^2 + 20*b5*t^3; % lateral acceleration 
    
    curvature = (dx*d2y - d2x*dy)/(dx^2 + dy^2)^(3/2); 
      
    
% elseif turn_signal == 2
%          
%  d2x = 1.4 ;
%  
%  duration = 2 ;
%  
%  curvature = 0;
 
else
     d2x = 0;
     d2y = 0;
    curvature=0;
    duration=0;
end

== matlab function TGASMODEL/Vehicle Dynamics and Environment(Actor and Sensor Simulation)/Pack Ego Actor ==
  data: pos input; a output Bus: BusActors1Actors size=1; vel input; yaw input; yawRate input
function a = packEgo(pos,vel,yaw,yawRate)
% Pack ego information into a single ego actor bus
%
% Imoprtant note:
% Output is a bus of type BusActorsActors. This is the same bus used by the
% Scenario Reader to output an individual actor. If you change the
% output bus name of Scenario Reader change the output bus name here
% as well by clicking on 'Edit Data' in the menu above.

a = struct(...
    'ActorID',1,...
    'Position', [pos(1) pos(2) 0], ...
    'Velocity', [vel(1) vel(2) 0], ...
    'Roll', 0, ...
    'Pitch', 0, ...
    'Yaw', yaw, ...
    'AngularVelocity', [0 0 yawRate]);

== stateflow chart TGASMODEL/Lanne Change Manoeuvre Planner/Decision Unit/Chart ==
  note: initial_lane = 0: right lane
      | initial_lane = 1: left lane
      | current_lane = 0: right lane
      | current_lane = 1: left lane
      | lead_car = 1: there is a lead car
      | lead_car = 0: there is no lead car
      | man_or_auto = 0: manual mode
      | man_or_auto = 1: autonomous mode
      | lane_changed = 1: the vehicle changed its lane after it starts to run.
      | lane_changed = 0: the vehicle hasn't changed its lane after it starts to run.
  state autonomous_mode
    state switch_left_lead_car
      entry:
      command = 1;
      lane_changed = 1;
    state go_straight_after_switch_left
      entry:
      command=0;
    state go_straight_before_switch_right
      entry:
      command=0;
    state switch_right_after_switch_left
      entry:
      command = 2;
    state lane_keeping
      entry:
      command = 0;
    state switch_right_lead_car
      entry:
      command = 2;
      lane_changed = 1;
    state switch_left_after_switch_right
      entry:
      command = 1;
    state go_straight_after_switch_right
      entry:
      command=0;
    state go_straight_before_switch_left
      entry:
      command = 0;
    go_straight_after_switch_left -> go_straight_before_switch_right [order 1] : after(4,sec)[lead_car==1&&current_lane ==1]
    switch_left_lead_car -> go_straight_after_switch_left : after(5,sec)
    go_straight_before_switch_right -> switch_right_after_switch_left : after(19,sec)
    switch_right_after_switch_left -> lane_keeping : after(6,sec)
    go_straight_after_switch_left -> lane_keeping [order 2] : after(5,sec)[lead_car == 1]
    lane_keeping -> switch_left_lead_car [order 2] : after(5,sec)[lead_car ==1&&consider_lane_changing==1&&can_lane_changing==1&&( current_lane ==0||(lane_changed == 0&&initial_lane==0))]
    (default) -> lane_keeping
    switch_left_after_switch_right -> lane_keeping : after(1,sec)
    lane_keeping -> switch_right_lead_car [order 1] : after(5,sec)[lead_car == 1&&consider_lane_changing==1 &&can_lane_changing==1&&( current_lane ==1||(lane_changed==0&&initial_lane==1))]
    go_straight_after_switch_right -> lane_keeping [order 2] : after(5,sec)[lead_car==1]
    go_straight_before_switch_left -> switch_left_after_switch_right : after(7,sec)
    switch_right_lead_car -> go_straight_after_switch_right : after(1,sec)
    go_straight_after_switch_right -> go_straight_before_switch_left [order 1] : after(5,sec)[lead_car==0&& current_lane ==0]
  (default) -> autonomous_mode
  data: command output; can_lane_changing input; consider_lane_changing input; lead_car input; initial_lane input; current_lane input; lane_changed local =0

== matlab function TGASMODEL/Lanne Change Manoeuvre Planner/Longitudinal Acceleration and steering decide/Steering Angle  ==
  data: turn_signal input; steering_lane_changing output; Steering_Angle input
function steering_lane_changing= straight_lane(turn_signal,Steering_Angle)

% This function outputs a certain steering angle with different turn_signal
% value.

% Input:
% turn_signal: a flag to indicate the vehicle's maneuver.

% Output:
% steering_curve_lane_changing_u_turn: steering angle for curve lane
% changing or u-turn.

if turn_signal == 1 
    % The vehicle will switch left in a curve lane with a steering angle
    % 0.1 rad.
    
    steering_lane_changing = -0.0872665;
    
elseif turn_signal ==2
    
    steering_lane_changing= 0.0872665;
    
else
    steering_lane_changing = Steering_Angle;
end

== stateflow chart TGASMODEL/Lanne Change Manoeuvre Planner/Decision Unit/Vehicle States ==
  note: command = 1, the vehicle switchs left,and turn_flag = 1.
      | command = 2, the vehicle switchs right,and turn_flag = 2.
      |
      | if vehicle keeps lane, turn_flag = 0.
      |
      | coor_trans_t is a time value which is used for coordinate transformation in
      | next subsystem:
      |
      | "Duration,Curvature and Longitudinal Acceleration calculation".
      |
      | initial_velocity_ego is the initial speed for the  maneuver
      |
      | current_lane = 0, the vehicle is at right lane.
      | current_lane = 1, the vehicle is at left lane
  state switch_right
    entry:
    turn_signal = 2;
    coor_trans_t = clock_time;
    initial_lane_changing_velocity_ego = longitudinal_velocity;
  state lane_keeping
    entry:
    turn_signal = 0;
  state switch_left
    entry:
    turn_signal = 1;
    coor_trans_t = clock_time;
    initial_lane_changing_velocity_ego = longitudinal_velocity;
  lane_keeping -> switch_right [order 1] : [command==2]
  switch_right -> lane_keeping : after(duration_lane_changing,sec){current_lane = 0;}
  (default) -> lane_keeping
  lane_keeping -> switch_left [order 2] : [command==1]
  switch_left -> lane_keeping : after(duration_lane_changing,sec){current_lane = 1;}
  data: turn_signal output; command input; clock_time input; coor_trans_t output; duration_lane_changing input; initial_lane_changing_velocity_ego output; current_lane output; longitudinal_velocity input

== matlab function TGASMODEL/Lanne Change Manoeuvre Planner/Longitudinal Acceleration and steering decide/Curve Lane or Not ==
  data: steeringLKA input; curve_lane_or_not output
function curve_lane_or_not  = is_curve_lane(steeringLKA)
% This function uses steering angle from LKA to judge whether the lane 
% curve is,so that the vehicle will use another algorithm to achieve curve 
% lane changing.

% Input:
% steeringLKA: steering angle from Lane Keeping Assist.

% Output:
% curve_lane_or_not: 0->not a curve lane,1->curve lane.

if abs(steeringLKA) >10^(-2.5)%(-2.8)
    curve_lane_or_not = 1;
else
    curve_lane_or_not = 0;
end
% if abs(steeringLKA) >10^(-3)||(abs(Curvature_1)>10^(-4)||abs(Curvature_)>10^(-4))
%     curve_lane_or_not = 1;
% else
%     curve_lane_or_not = 0;
% end
